simulink model "CL3_prob3_v2"  (R2014a)
settings: Solver=ode45  StartTime=0.0  StopTime=800  RelTol=1e-9
values from neighbouring files (symbols this model uses):
  a1 = 6.67    [CL3_insulin_glucose_model_student.m]
  alph = 7.5    [CL3_insulin_glucose_model_student.m]
  bet = 1.77    [CL3_insulin_glucose_model_student.m]
  C1 = 300    [CL3_insulin_glucose_model_student.m]
  C2 = 144    [CL3_insulin_glucose_model_student.m]
  C3 = 100    [CL3_insulin_glucose_model_student.m]
  C5 = 26    [CL3_insulin_glucose_model_student.m]
  E = 0.2    [CL3_insulin_glucose_model_student.m]
  k = (1/C4)*(1/Vi+1/(E*ti))    (= 0.00176136363636)    [CL3_insulin_glucose_model_student.m]
  Rg = 180    [CL3_insulin_glucose_model_student.m]
  Rm = 209    [CL3_insulin_glucose_model_student.m]
  ti = 100    [CL3_insulin_glucose_model_student.m]
  tp = 6    [CL3_insulin_glucose_model_student.m]
  Ub = 72    [CL3_insulin_glucose_model_student.m]
  Um = 94    [CL3_insulin_glucose_model_student.m]
  Uo = 4    [CL3_insulin_glucose_model_student.m]
  Vg = 10    [CL3_insulin_glucose_model_student.m]
  Vi = 11    [CL3_insulin_glucose_model_student.m]
  Vp = 3    [CL3_insulin_glucose_model_student.m]
settings Model: Creator=widderp  LastModifiedBy=widderp

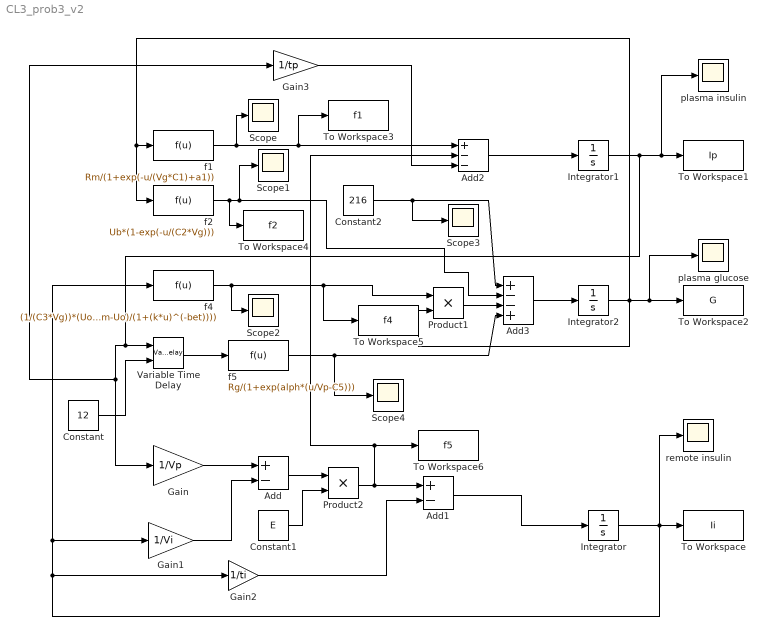
== system CL3_prob3_v2 ==
  Add : Sum  Inputs=+-
  Add1 : Sum  Inputs=+-
  Add2 : Sum  Inputs=+--
  Add3 : Sum  Inputs=+--+
  Constant : Constant  Value=12
  Constant1 : Constant  Value=E
  Constant2 : Constant  Value=216
  Gain : Gain  Gain=1/Vp
  Gain1 : Gain  Gain=1/Vi
  Gain2 : Gain  Gain=1/ti
  Gain3 : Gain  Gain=1/tp
  Integrator : Integrator  InitialCondition=160
  Integrator1 : Integrator  InitialCondition=60
  Integrator2 : Integrator  InitialCondition=12000
  Product1 : Product
  Product2 : Product
  Scope{,1..4} (5 alike) : Scope
      Scope settings: YMin=0  YMax=160  SaveName=ScopeData4
      Scope1 settings: SaveName=ScopeData5
      Scope2 settings: SaveName=ScopeData6
      Scope3 settings: SaveName=ScopeData3
      Scope4 settings: SaveName=ScopeData7
  To Workspace : ToWorkspace  VariableName=Ii  SampleTime=-1
  To Workspace1 : ToWorkspace  VariableName=Ip  SampleTime=-1
  To Workspace2 : ToWorkspace  VariableName=G  SampleTime=-1
  To Workspace3 : ToWorkspace  VariableName=f1  SampleTime=-1
  To Workspace4 : ToWorkspace  VariableName=f2  SampleTime=-1
  To Workspace5 : ToWorkspace  VariableName=f4  SampleTime=-1
  To Workspace6 : ToWorkspace  VariableName=f5  SampleTime=-1
  Variable Time Delay : VariableTransportDelay  VariableDelayType=Variable transport delay  MaximumDelay=5000
  f1 : Fcn  Expr=Rm/(1+exp(-u/(Vg*C1)+a1))
  f2 : Fcn  Expr=Ub*(1-exp(-u/(C2*Vg)))
  f4 : Fcn  Expr=(1/(C3*Vg))*(Uo+((Um-Uo)/(1+(k*u)^(-bet))))
  f5 : Fcn  Expr=Rg/(1+exp(alph*(u/Vp-C5)))
  plasma glucose : Scope
      settings: YMin=0  YMax=15000
  plasma insulin : Scope
      settings: YMin=10  YMax=130
  remote insulin : Scope
      settings: YMin=157.5  YMax=180  SaveName=ScopeData2
  wires:
  Integrator/1 -> remote insulin/1, Gain2/1, Gain1/1, f4/1, To Workspace/1
  Integrator2/1 -> Product1/2, f2/1, f1/1, plasma glucose/1, To Workspace2/1
  Variable Time Delay/1 -> f5/1
  Integrator1/1 -> Gain/1, Gain3/1, Variable Time Delay/1, plasma insulin/1, To Workspace1/1
  Constant/1 -> Variable Time Delay/2
  Constant1/1 -> Product2/2
  Add/1 -> Product2/1
  Gain/1 -> Add/1
  Gain1/1 -> Add/2
  Product2/1 -> To Workspace6/1, Add2/2, Add1/1
  Gain2/1 -> Add1/2
  Add1/1 -> Integrator/1
  f1/1 -> Scope/1, To Workspace3/1, Add2/1
  Gain3/1 -> Add2/3
  Add2/1 -> Integrator1/1
  Constant2/1 -> Scope3/1, Add3/1
  f2/1 -> To Workspace4/1, Scope1/1, Add3/2
  Add3/1 -> Integrator2/1
  f4/1 -> To Workspace5/1, Product1/1, Scope2/1
  f5/1 -> Scope4/1, Add3/4
  Product1/1 -> Add3/3
